simulink subsystem "Modes"  (R2022a)
settings: Solver=VariableStepAuto  StartTime=0.0  StopTime=10.0  RelTol=1e-3
settings Model: Creator=ivanl  LastModifiedBy=ivanl

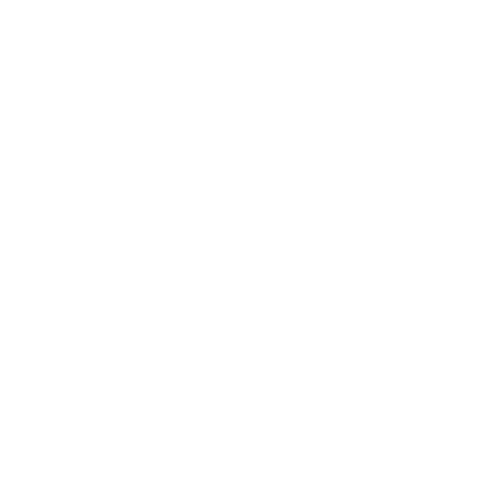
[thumbnail: Simulink's stored preview of the top-level diagram]
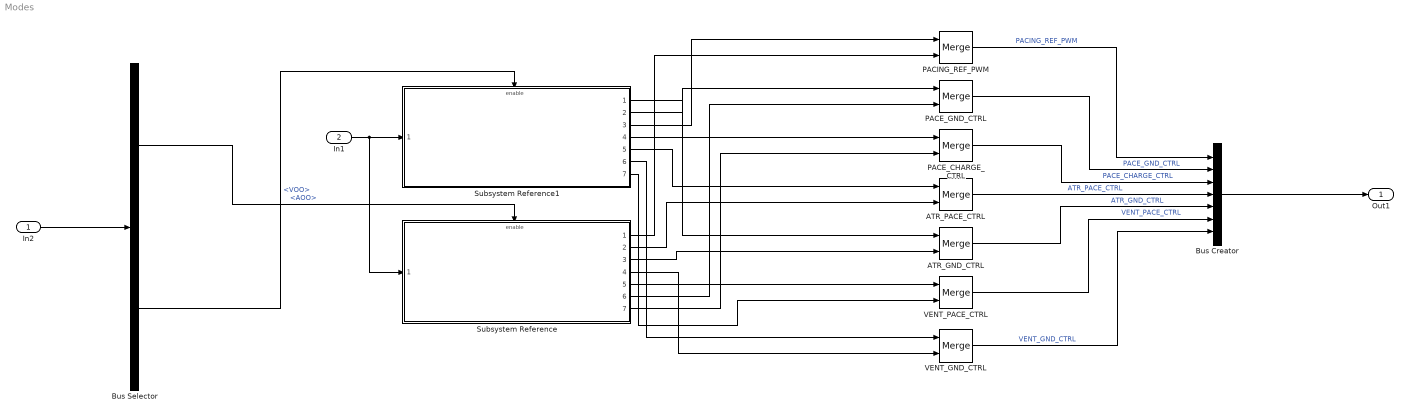
== system Modes ==
  In2 : Inport
  In1 : Inport  Port=2
  ATR_GND_CTRL : Merge
  ATR_PACE_CTRL : Merge
  Bus Creator : BusCreator  Inputs=7
  Bus Selector : BusSelector  OutputSignals=AOO,VOO
  PACE_CHARGE_CTRL : Merge
  PACE_GND_CTRL : Merge
  PACING_REF_PWM : Merge
  Subsystem Reference : Subsystem  ReferencedSubsystem=AOO_mode
  Subsystem Reference1 : Subsystem  ReferencedSubsystem=VOO_mode
  VENT_GND_CTRL : Merge
  VENT_PACE_CTRL : Merge
  Out1 : Outport
  wires:
  Subsystem Reference1/3 -> PACING_REF_PWM/1
  Subsystem Reference/1 -> PACING_REF_PWM/2
  Subsystem Reference1/2 -> PACE_GND_CTRL/1
  Subsystem Reference/6 -> PACE_GND_CTRL/2
  Subsystem Reference/7 -> PACE_CHARGE_CTRL/2
  Subsystem Reference1/1 -> PACE_CHARGE_CTRL/1
  Subsystem Reference1/5 -> ATR_PACE_CTRL/1
  Subsystem Reference/2 -> ATR_PACE_CTRL/2
  Subsystem Reference1/4 -> ATR_GND_CTRL/1
  Subsystem Reference/3 -> ATR_GND_CTRL/2
  Subsystem Reference/5 -> VENT_PACE_CTRL/1
  Subsystem Reference1/7 -> VENT_PACE_CTRL/2
  Subsystem Reference1/6 -> VENT_GND_CTRL/1
  Subsystem Reference/4 -> VENT_GND_CTRL/2
  PACING_REF_PWM/1 -> Bus Creator/1  "PACING_REF_PWM"
  PACE_GND_CTRL/1 -> Bus Creator/2  "PACE_GND_CTRL"
  PACE_CHARGE_CTRL/1 -> Bus Creator/3  "PACE_CHARGE_CTRL"
  ATR_PACE_CTRL/1 -> Bus Creator/4  "ATR_PACE_CTRL"
  ATR_GND_CTRL/1 -> Bus Creator/5  "ATR_GND_CTRL"
  VENT_PACE_CTRL/1 -> Bus Creator/6  "VENT_PACE_CTRL"
  VENT_GND_CTRL/1 -> Bus Creator/7  "VENT_GND_CTRL"
  Bus Creator/1 -> Out1/1
  In2/1 -> Bus Selector/1
  Bus Selector/1 -> Subsystem Reference/Enable  "<AOO>"
  Bus Selector/2 -> Subsystem Reference1/Enable  "<VOO>"
  In1/1 -> Subsystem Reference1/1, Subsystem Reference/1
